simulink model "lab1"  (R2016b)
settings: Solver=FixedStepDiscrete  StartTime=0.0  StopTime=5  RelTol=1e-3  EnableMultiTasking=on
libraries: simulink x1
settings Model: SimulationMode=external  Creator=tommy  LastModifiedBy=johhel16
settings SolverCC: PositivePriorityOrder=on
settings OptimizationCC: LifeSpan=1  MaxStackSize=64
settings DebuggingCC: SFUnexpectedBacktrackingDiag=warning  SFNoUnconditionalDefaultTransitionDiag=warning  SFExecutionAtInitializationDiag=none
settings HardwareCC: ProdBitPerPointer=32  ProdBitPerSizeT=32  ProdBitPerPtrDiffT=32  ProdLargestAtomicInteger=Long  ProdLargestAtomicFloat=Double  ProdWordSize=32  ProdHWDeviceType=ARM Compatible->ARM Cortex
settings RTWCC: SystemTargetFile=ert.tlc  HardwareBoard=Raspberry Pi  TLCOptions=-aInlineSetEventsForThisBaseRateFcn=TLC_FALSE -aSuppressMultiTaskScheduler=TLC_FALSE -aRateBasedStepFcn=0  TemplateMakefile=ert_default_tmf  Description=Embedded Coder  Toolchain=GNU GCC Raspberry Pi
settings CodeAppCC: ForceParamTrailComments=on  IgnoreCustomStorageClasses=off  OperatorAnnotations=on  SimulinkDataObjDesc=on  SFDataObjDesc=on  MATLABFcnDesc=on  InsertBlockDesc=on  MATLABSourceComments=on
settings ERTTargetCC: SupportVariableSizeSignals=on
settings ConfigComp: CovMetricSettings=dw  CovHtmlReporting=on  CovSaveCumulativeToWorkspaceVar=on  CovSaveSingleToWorkspaceVar=on  CovExternalEMLEnable=off

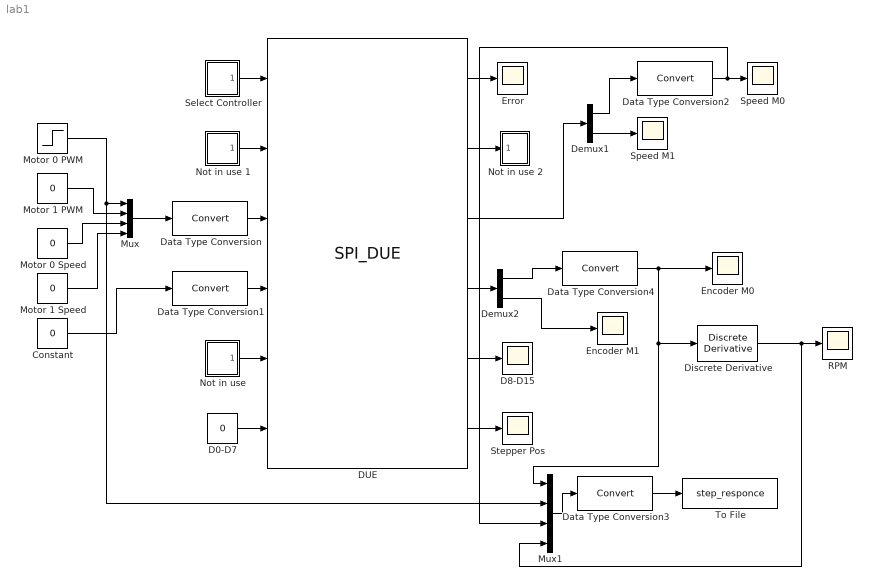
== system lab1 ==
  Constant : Constant  Value=0
  D0-D7 : Constant  Value=0  OutDataTypeStr=uint8
  D8-D15 : Scope
  DUE : S-Function  InitFcn=try, set_param(gcb,'FunctionName','SPI_DUE'), end  FunctionName=SPI_DUE  Parameters=uint8(1),uint32(4000000)  SFunctionModules=SPI_DUE_wrapper  SFunctionDeploymentMode=off  EnableBusSupport=off  mask(S-Function Builder){}
      mask help: Simulink:masks:SFunctionBuilder_MD
      mask init:
      | val = [[.9  0.75 0.75 1 1 .9 .9 1]',[1 1 0.75 0.75 .9 .9 1 .9]'];try , sys = get_param(gcb,'SfunBuilderFcnName');if isempty(sys), sys = get_param(gcb,'FunctionName'); end,catch, sys = get_param(gcb,'FunctionName'); end
      settings: CopyFcn=set_param(gcbh,'LinkStatus','none')  PreSaveFcn=try, set_param(gcb,'FunctionName','SPI_DUE'), end  OpenFcn=sfunctionwizard(gcbh)
      mask Display: plot(val(:,1),val(:,2)),disp(sys), port_label('input',1,'Select'), port_label('input',2,'Sample_Time'), port_label('input',3,'Set_Speed_DC'), port_label('input',4,'Set_Speed_Stepper'), port_label('input',5,'Controllers'), port_label('input',6,'Set_Digital'), port_label('output',1,'Status'), port_label('output',2,'Current'), port_label('output',3,'Motor_Speed'), port_label('output',4,'Motor_Encoder'), port_label('output',5,'Read_Digital'), port_label('output',6,'Stepper_Pos')
  Data Type Conversion{,1..4} (5 alike) : DataTypeConversion
  Demux1 : Demux  Outputs=2
  Demux2 : Demux  Outputs=2
  Discrete Derivative : simulink/Discrete/Discrete Derivative  gainval=60/512  ICPrevScaledInput=0.0  OutMin=[]  OutMax=[]  OutDataType=fixdt(1, 16)  OutScaling=2^-10  DoSatur=off
  Encoder M0 : Scope
  Encoder M1 : Scope
  Error : Scope
  Motor 0 PWM : Step  After=568  SampleTime=0.002
  Motor 0 Speed : Constant  Value=0
  Motor 1 PWM : Constant  Value=0
  Motor 1 Speed : Constant  Value=0
  Mux : Mux
  Mux1 : Mux
  Not in use : Subsystem
  Not in use 1 : Subsystem
  Not in use 2 : Subsystem
  RPM : Scope
  Select Controller : Subsystem
  Speed M0 : Scope
  Speed M1 : Scope
  Stepper Pos : Scope
  To File : ToFile  Filename=step_responce
  wires:
  Mux/1 -> Data Type Conversion/1
  DUE/1 -> Error/1
  Data Type Conversion/1 -> DUE/3
  Demux2/2 -> Encoder M1/1
  DUE/5 -> D8-D15/1
  DUE/4 -> Demux2/1
  Not in use 1/1(Out1) -> DUE/2
  Select Controller/1(Out1) -> DUE/1
  DUE/2 -> Not in use 2/1(In1)
  DUE/3 -> Demux1/1
  Not in use/1(Out1) -> DUE/5
  Data Type Conversion3/1 -> To File/1
  Motor 1 Speed/1 -> Mux/4
  Demux2/1 -> Data Type Conversion4/1
  DUE/6 -> Stepper Pos/1
  D0-D7/1 -> DUE/6
  Data Type Conversion1/1 -> DUE/4
  Demux1/2 -> Speed M1/1
  Demux1/1 -> Data Type Conversion2/1
  Data Type Conversion2/1 -> Mux1/3, Speed M0/1
  Constant/1 -> Data Type Conversion1/1
  Motor 0 PWM/1 -> Mux1/2, Mux/1
  Motor 1 PWM/1 -> Mux/2
  Motor 0 Speed/1 -> Mux/3
  Mux1/1 -> Data Type Conversion3/1
  Data Type Conversion4/1 -> Encoder M0/1, Discrete Derivative/1, Mux1/1
  Discrete Derivative/1 -> Mux1/4, RPM/1

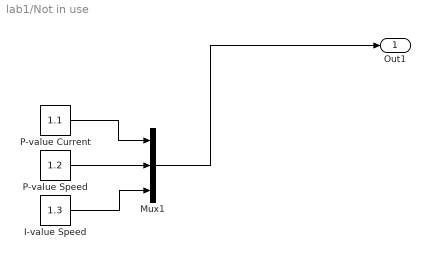
== system lab1/Not in use ==
  I-value Speed : Constant  Value=1.3  OutDataTypeStr=single
  Mux1 : Mux  Inputs=3
  P-value Current : Constant  Value=1.1  OutDataTypeStr=single
  P-value Speed : Constant  Value=1.2  OutDataTypeStr=single
  Out1 : Outport
  wires:
  Mux1/1 -> Out1/1
  P-value Current/1 -> Mux1/1
  I-value Speed/1 -> Mux1/3
  P-value Speed/1 -> Mux1/2

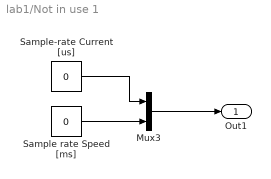
== system lab1/Not in use 1 ==
  Mux3 : Mux  Inputs=2
  Sample rate Speed [ms] : Constant  Value=0  OutDataTypeStr=uint16
  Sample-rate Current [us] : Constant  Value=0  OutDataTypeStr=uint16
  Out1 : Outport
  wires:
  Sample-rate Current [us]/1 -> Mux3/1
  Mux3/1 -> Out1/1
  Sample rate Speed [ms]/1 -> Mux3/2

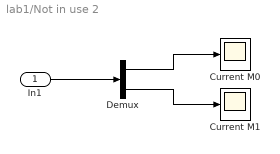
== system lab1/Not in use 2 ==
  In1 : Inport
  Current M0 : Scope
  Current M1 : Scope
  Demux : Demux  Outputs=2
  wires:
  In1/1 -> Demux/1
  Demux/2 -> Current M1/1
  Demux/1 -> Current M0/1

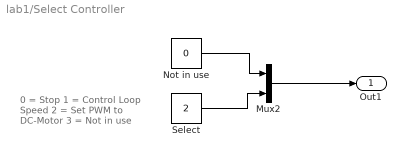
== system lab1/Select Controller ==
  note: 0 = Stop
      | 1 = Control Loop Speed
      | 2 = Set PWM to DC-Motor
      | 3 = Not in use
  Mux2 : Mux  Inputs=2
  Not in use : Constant  Value=0  OutDataTypeStr=uint8
  Select : Constant  Value=2  OutDataTypeStr=uint8
  Out1 : Outport
  wires:
  Select/1 -> Mux2/2
  Not in use/1 -> Mux2/1
  Mux2/1 -> Out1/1
